simulink model "Filter"  (R2017b)
settings: Solver=VariableStepAuto  StartTime=0.0  StopTime=10  RelTol=1e-3
undefined symbols (not defined in the file or in its folder): designMultirateFIR
libraries: dspsrcs4 x2, dspmlti4 x1
(part 2 of 3)

== system Filter/HighpassH/Resonator132 ==
  In1 : Inport
  Delay : Delay  DelayLength=1
  Gain : Gain  Gain=-0.3143-0.94932i
  GainH : Gain  Gain=-0.57421+0.81871i
  Sum1 : Sum  Inputs=|++
  Out1 : Outport
  wires:
  In1/1 -> Sum1/1
  GainH/1 -> Out1/1
  Gain/1 -> Sum1/2
  Delay/1 -> Gain/1
  Sum1/1 -> Delay/1, GainH/1

== system Filter/HighpassH/Resonator133 ==
  In1 : Inport
  Delay : Delay  DelayLength=1
  Gain : Gain  Gain=-0.28779-0.95769i
  GainH : Gain  Gain=0.58553-0.81065i
  Sum1 : Sum  Inputs=|++
  Out1 : Outport
  wires:
  In1/1 -> Sum1/1
  GainH/1 -> Out1/1
  Gain/1 -> Sum1/2
  Delay/1 -> Gain/1
  Sum1/1 -> Delay/1, GainH/1

== system Filter/HighpassH/Resonator134 ==
  In1 : Inport
  Delay : Delay  DelayLength=1
  Gain : Gain  Gain=-0.26106-0.96532i
  GainH : Gain  Gain=-0.59675+0.80243i
  Sum1 : Sum  Inputs=|++
  Out1 : Outport
  wires:
  In1/1 -> Sum1/1
  GainH/1 -> Out1/1
  Gain/1 -> Sum1/2
  Delay/1 -> Gain/1
  Sum1/1 -> Delay/1, GainH/1

== system Filter/HighpassH/Resonator135 ==
  In1 : Inport
  Delay : Delay  DelayLength=1
  Gain : Gain  Gain=-0.23412-0.97221i
  GainH : Gain  Gain=0.60784-0.79406i
  Sum1 : Sum  Inputs=|++
  Out1 : Outport
  wires:
  In1/1 -> Sum1/1
  GainH/1 -> Out1/1
  Gain/1 -> Sum1/2
  Delay/1 -> Gain/1
  Sum1/1 -> Delay/1, GainH/1

== system Filter/HighpassH/Resonator136 ==
  In1 : Inport
  Delay : Delay  DelayLength=1
  Gain : Gain  Gain=-0.20701-0.97834i
  GainH : Gain  Gain=-0.61882+0.78553i
  Sum1 : Sum  Inputs=|++
  Out1 : Outport
  wires:
  In1/1 -> Sum1/1
  GainH/1 -> Out1/1
  Gain/1 -> Sum1/2
  Delay/1 -> Gain/1
  Sum1/1 -> Delay/1, GainH/1

== system Filter/HighpassH/Resonator137 ==
  In1 : Inport
  Delay : Delay  DelayLength=1
  Gain : Gain  Gain=-0.17973-0.98372i
  GainH : Gain  Gain=0.62968-0.77685i
  Sum1 : Sum  Inputs=|++
  Out1 : Outport
  wires:
  In1/1 -> Sum1/1
  GainH/1 -> Out1/1
  Gain/1 -> Sum1/2
  Delay/1 -> Gain/1
  Sum1/1 -> Delay/1, GainH/1

== system Filter/HighpassH/Resonator138 ==
  In1 : Inport
  Delay : Delay  DelayLength=1
  Gain : Gain  Gain=-0.15231-0.98833i
  GainH : Gain  Gain=-0.64042+0.76803i
  Sum1 : Sum  Inputs=|++
  Out1 : Outport
  wires:
  In1/1 -> Sum1/1
  GainH/1 -> Out1/1
  Gain/1 -> Sum1/2
  Delay/1 -> Gain/1
  Sum1/1 -> Delay/1, GainH/1

== system Filter/HighpassH/Resonator139 ==
  In1 : Inport
  Delay : Delay  DelayLength=1
  Gain : Gain  Gain=-0.12478-0.99218i
  GainH : Gain  Gain=0.65103-0.75905i
  Sum1 : Sum  Inputs=|++
  Out1 : Outport
  wires:
  In1/1 -> Sum1/1
  GainH/1 -> Out1/1
  Gain/1 -> Sum1/2
  Delay/1 -> Gain/1
  Sum1/1 -> Delay/1, GainH/1

== system Filter/HighpassH/Resonator14 ==
  In1 : Inport
  Delay : Delay  DelayLength=1
  Gain : Gain  Gain=0.44281+0.89662i
  GainH : Gain  Gain=-0.85661-0.51596i
  Sum1 : Sum  Inputs=|++
  Out1 : Outport
  wires:
  In1/1 -> Sum1/1
  GainH/1 -> Out1/1
  Gain/1 -> Sum1/2
  Delay/1 -> Gain/1
  Sum1/1 -> Delay/1, GainH/1

== system Filter/HighpassH/Resonator140 ==
  In1 : Inport
  Delay : Delay  DelayLength=1
  Gain : Gain  Gain=-0.097152-0.99527i
  GainH : Gain  Gain=-0.66152+0.74993i
  Sum1 : Sum  Inputs=|++
  Out1 : Outport
  wires:
  In1/1 -> Sum1/1
  GainH/1 -> Out1/1
  Gain/1 -> Sum1/2
  Delay/1 -> Gain/1
  Sum1/1 -> Delay/1, GainH/1

== system Filter/HighpassH/Resonator141 ==
  In1 : Inport
  Delay : Delay  DelayLength=1
  Gain : Gain  Gain=-0.069448-0.99759i
  GainH : Gain  Gain=0.67188-0.74066i
  Sum1 : Sum  Inputs=|++
  Out1 : Outport
  wires:
  In1/1 -> Sum1/1
  GainH/1 -> Out1/1
  Gain/1 -> Sum1/2
  Delay/1 -> Gain/1
  Sum1/1 -> Delay/1, GainH/1

== system Filter/HighpassH/Resonator142 ==
  In1 : Inport
  Delay : Delay  DelayLength=1
  Gain : Gain  Gain=-0.04169-0.99913i
  GainH : Gain  Gain=-0.68211+0.73125i
  Sum1 : Sum  Inputs=|++
  Out1 : Outport
  wires:
  In1/1 -> Sum1/1
  GainH/1 -> Out1/1
  Gain/1 -> Sum1/2
  Delay/1 -> Gain/1
  Sum1/1 -> Delay/1, GainH/1

== system Filter/HighpassH/Resonator143 ==
  In1 : Inport
  Delay : Delay  DelayLength=1
  Gain : Gain  Gain=-0.0139-0.9999i
  GainH : Gain  Gain=0.69221-0.7217i
  Sum1 : Sum  Inputs=|++
  Out1 : Outport
  wires:
  In1/1 -> Sum1/1
  GainH/1 -> Out1/1
  Gain/1 -> Sum1/2
  Delay/1 -> Gain/1
  Sum1/1 -> Delay/1, GainH/1

== system Filter/HighpassH/Resonator144 ==
  In1 : Inport
  Delay : Delay  DelayLength=1
  Gain : Gain  Gain=0.0139-0.9999i
  GainH : Gain  Gain=-0.70218+0.712i
  Sum1 : Sum  Inputs=|++
  Out1 : Outport
  wires:
  In1/1 -> Sum1/1
  GainH/1 -> Out1/1
  Gain/1 -> Sum1/2
  Delay/1 -> Gain/1
  Sum1/1 -> Delay/1, GainH/1

== system Filter/HighpassH/Resonator145 ==
  In1 : Inport
  Delay : Delay  DelayLength=1
  Gain : Gain  Gain=0.04169-0.99913i
  GainH : Gain  Gain=0.712-0.70218i
  Sum1 : Sum  Inputs=|++
  Out1 : Outport
  wires:
  In1/1 -> Sum1/1
  GainH/1 -> Out1/1
  Gain/1 -> Sum1/2
  Delay/1 -> Gain/1
  Sum1/1 -> Delay/1, GainH/1

== system Filter/HighpassH/Resonator146 ==
  In1 : Inport
  Delay : Delay  DelayLength=1
  Gain : Gain  Gain=0.069448-0.99759i
  GainH : Gain  Gain=-0.7217+0.69221i
  Sum1 : Sum  Inputs=|++
  Out1 : Outport
  wires:
  In1/1 -> Sum1/1
  GainH/1 -> Out1/1
  Gain/1 -> Sum1/2
  Delay/1 -> Gain/1
  Sum1/1 -> Delay/1, GainH/1

== system Filter/HighpassH/Resonator147 ==
  In1 : Inport
  Delay : Delay  DelayLength=1
  Gain : Gain  Gain=0.097152-0.99527i
  GainH : Gain  Gain=0.73125-0.68211i
  Sum1 : Sum  Inputs=|++
  Out1 : Outport
  wires:
  In1/1 -> Sum1/1
  GainH/1 -> Out1/1
  Gain/1 -> Sum1/2
  Delay/1 -> Gain/1
  Sum1/1 -> Delay/1, GainH/1

== system Filter/HighpassH/Resonator148 ==
  In1 : Inport
  Delay : Delay  DelayLength=1
  Gain : Gain  Gain=0.12478-0.99218i
  GainH : Gain  Gain=-0.74066+0.67188i
  Sum1 : Sum  Inputs=|++
  Out1 : Outport
  wires:
  In1/1 -> Sum1/1
  GainH/1 -> Out1/1
  Gain/1 -> Sum1/2
  Delay/1 -> Gain/1
  Sum1/1 -> Delay/1, GainH/1

== system Filter/HighpassH/Resonator149 ==
  In1 : Inport
  Delay : Delay  DelayLength=1
  Gain : Gain  Gain=0.15231-0.98833i
  GainH : Gain  Gain=0.74993-0.66152i
  Sum1 : Sum  Inputs=|++
  Out1 : Outport
  wires:
  In1/1 -> Sum1/1
  GainH/1 -> Out1/1
  Gain/1 -> Sum1/2
  Delay/1 -> Gain/1
  Sum1/1 -> Delay/1, GainH/1

== system Filter/HighpassH/Resonator15 ==
  In1 : Inport
  Delay : Delay  DelayLength=1
  Gain : Gain  Gain=0.41771+0.90858i
  GainH : Gain  Gain=0.84936+0.52782i
  Sum1 : Sum  Inputs=|++
  Out1 : Outport
  wires:
  In1/1 -> Sum1/1
  GainH/1 -> Out1/1
  Gain/1 -> Sum1/2
  Delay/1 -> Gain/1
  Sum1/1 -> Delay/1, GainH/1

== system Filter/HighpassH/Resonator150 ==
  In1 : Inport
  Delay : Delay  DelayLength=1
  Gain : Gain  Gain=0.17973-0.98372i
  GainH : Gain  Gain=-0.75905+0.65103i
  Sum1 : Sum  Inputs=|++
  Out1 : Outport
  wires:
  In1/1 -> Sum1/1
  GainH/1 -> Out1/1
  Gain/1 -> Sum1/2
  Delay/1 -> Gain/1
  Sum1/1 -> Delay/1, GainH/1

== system Filter/HighpassH/Resonator151 ==
  In1 : Inport
  Delay : Delay  DelayLength=1
  Gain : Gain  Gain=0.20701-0.97834i
  GainH : Gain  Gain=0.76803-0.64042i
  Sum1 : Sum  Inputs=|++
  Out1 : Outport
  wires:
  In1/1 -> Sum1/1
  GainH/1 -> Out1/1
  Gain/1 -> Sum1/2
  Delay/1 -> Gain/1
  Sum1/1 -> Delay/1, GainH/1

== system Filter/HighpassH/Resonator152 ==
  In1 : Inport
  Delay : Delay  DelayLength=1
  Gain : Gain  Gain=0.23412-0.97221i
  GainH : Gain  Gain=-0.77685+0.62968i
  Sum1 : Sum  Inputs=|++
  Out1 : Outport
  wires:
  In1/1 -> Sum1/1
  GainH/1 -> Out1/1
  Gain/1 -> Sum1/2
  Delay/1 -> Gain/1
  Sum1/1 -> Delay/1, GainH/1

== system Filter/HighpassH/Resonator153 ==
  In1 : Inport
  Delay : Delay  DelayLength=1
  Gain : Gain  Gain=0.26106-0.96532i
  GainH : Gain  Gain=0.78553-0.61882i
  Sum1 : Sum  Inputs=|++
  Out1 : Outport
  wires:
  In1/1 -> Sum1/1
  GainH/1 -> Out1/1
  Gain/1 -> Sum1/2
  Delay/1 -> Gain/1
  Sum1/1 -> Delay/1, GainH/1

== system Filter/HighpassH/Resonator154 ==
  In1 : Inport
  Delay : Delay  DelayLength=1
  Gain : Gain  Gain=0.28779-0.95769i
  GainH : Gain  Gain=-0.79406+0.60784i
  Sum1 : Sum  Inputs=|++
  Out1 : Outport
  wires:
  In1/1 -> Sum1/1
  GainH/1 -> Out1/1
  Gain/1 -> Sum1/2
  Delay/1 -> Gain/1
  Sum1/1 -> Delay/1, GainH/1

== system Filter/HighpassH/Resonator155 ==
  In1 : Inport
  Delay : Delay  DelayLength=1
  Gain : Gain  Gain=0.3143-0.94932i
  GainH : Gain  Gain=0.80243-0.59675i
  Sum1 : Sum  Inputs=|++
  Out1 : Outport
  wires:
  In1/1 -> Sum1/1
  GainH/1 -> Out1/1
  Gain/1 -> Sum1/2
  Delay/1 -> Gain/1
  Sum1/1 -> Delay/1, GainH/1

== system Filter/HighpassH/Resonator156 ==
  In1 : Inport
  Delay : Delay  DelayLength=1
  Gain : Gain  Gain=0.34057-0.94022i
  GainH : Gain  Gain=-0.81065+0.58553i
  Sum1 : Sum  Inputs=|++
  Out1 : Outport
  wires:
  In1/1 -> Sum1/1
  GainH/1 -> Out1/1
  Gain/1 -> Sum1/2
  Delay/1 -> Gain/1
  Sum1/1 -> Delay/1, GainH/1

== system Filter/HighpassH/Resonator157 ==
  In1 : Inport
  Delay : Delay  DelayLength=1
  Gain : Gain  Gain=0.36657-0.93039i
  GainH : Gain  Gain=0.81871-0.57421i
  Sum1 : Sum  Inputs=|++
  Out1 : Outport
  wires:
  In1/1 -> Sum1/1
  GainH/1 -> Out1/1
  Gain/1 -> Sum1/2
  Delay/1 -> Gain/1
  Sum1/1 -> Delay/1, GainH/1

== system Filter/HighpassH/Resonator158 ==
  In1 : Inport
  Delay : Delay  DelayLength=1
  Gain : Gain  Gain=0.39229-0.91984i
  GainH : Gain  Gain=-0.82661+0.56277i
  Sum1 : Sum  Inputs=|++
  Out1 : Outport
  wires:
  In1/1 -> Sum1/1
  GainH/1 -> Out1/1
  Gain/1 -> Sum1/2
  Delay/1 -> Gain/1
  Sum1/1 -> Delay/1, GainH/1

== system Filter/HighpassH/Resonator159 ==
  In1 : Inport
  Delay : Delay  DelayLength=1
  Gain : Gain  Gain=0.41771-0.90858i
  GainH : Gain  Gain=0.83435-0.55123i
  Sum1 : Sum  Inputs=|++
  Out1 : Outport
  wires:
  In1/1 -> Sum1/1
  GainH/1 -> Out1/1
  Gain/1 -> Sum1/2
  Delay/1 -> Gain/1
  Sum1/1 -> Delay/1, GainH/1

== system Filter/HighpassH/Resonator16 ==
  In1 : Inport
  Delay : Delay  DelayLength=1
  Gain : Gain  Gain=0.39229+0.91984i
  GainH : Gain  Gain=-0.84194-0.53958i
  Sum1 : Sum  Inputs=|++
  Out1 : Outport
  wires:
  In1/1 -> Sum1/1
  GainH/1 -> Out1/1
  Gain/1 -> Sum1/2
  Delay/1 -> Gain/1
  Sum1/1 -> Delay/1, GainH/1

== system Filter/HighpassH/Resonator160 ==
  In1 : Inport
  Delay : Delay  DelayLength=1
  Gain : Gain  Gain=0.44281-0.89662i
  GainH : Gain  Gain=-0.84194+0.53958i
  Sum1 : Sum  Inputs=|++
  Out1 : Outport
  wires:
  In1/1 -> Sum1/1
  GainH/1 -> Out1/1
  Gain/1 -> Sum1/2
  Delay/1 -> Gain/1
  Sum1/1 -> Delay/1, GainH/1

== system Filter/HighpassH/Resonator161 ==
  In1 : Inport
  Delay : Delay  DelayLength=1
  Gain : Gain  Gain=0.46756-0.88396i
  GainH : Gain  Gain=0.84936-0.52782i
  Sum1 : Sum  Inputs=|++
  Out1 : Outport
  wires:
  In1/1 -> Sum1/1
  GainH/1 -> Out1/1
  Gain/1 -> Sum1/2
  Delay/1 -> Gain/1
  Sum1/1 -> Delay/1, GainH/1

== system Filter/HighpassH/Resonator162 ==
  In1 : Inport
  Delay : Delay  DelayLength=1
  Gain : Gain  Gain=0.49195-0.87062i
  GainH : Gain  Gain=-0.85661+0.51596i
  Sum1 : Sum  Inputs=|++
  Out1 : Outport
  wires:
  In1/1 -> Sum1/1
  GainH/1 -> Out1/1
  Gain/1 -> Sum1/2
  Delay/1 -> Gain/1
  Sum1/1 -> Delay/1, GainH/1

== system Filter/HighpassH/Resonator163 ==
  In1 : Inport
  Delay : Delay  DelayLength=1
  Gain : Gain  Gain=0.51596-0.85661i
  GainH : Gain  Gain=0.8637-0.50401i
  Sum1 : Sum  Inputs=|++
  Out1 : Outport
  wires:
  In1/1 -> Sum1/1
  GainH/1 -> Out1/1
  Gain/1 -> Sum1/2
  Delay/1 -> Gain/1
  Sum1/1 -> Delay/1, GainH/1

== system Filter/HighpassH/Resonator164 ==
  In1 : Inport
  Delay : Delay  DelayLength=1
  Gain : Gain  Gain=0.53958-0.84194i
  GainH : Gain  Gain=-0.87062+0.49195i
  Sum1 : Sum  Inputs=|++
  Out1 : Outport
  wires:
  In1/1 -> Sum1/1
  GainH/1 -> Out1/1
  Gain/1 -> Sum1/2
  Delay/1 -> Gain/1
  Sum1/1 -> Delay/1, GainH/1

== system Filter/HighpassH/Resonator165 ==
  In1 : Inport
  Delay : Delay  DelayLength=1
  Gain : Gain  Gain=0.56277-0.82661i
  GainH : Gain  Gain=0.87738-0.4798i
  Sum1 : Sum  Inputs=|++
  Out1 : Outport
  wires:
  In1/1 -> Sum1/1
  GainH/1 -> Out1/1
  Gain/1 -> Sum1/2
  Delay/1 -> Gain/1
  Sum1/1 -> Delay/1, GainH/1

== system Filter/HighpassH/Resonator166 ==
  In1 : Inport
  Delay : Delay  DelayLength=1
  Gain : Gain  Gain=0.58553-0.81065i
  GainH : Gain  Gain=-0.88396+0.46756i
  Sum1 : Sum  Inputs=|++
  Out1 : Outport
  wires:
  In1/1 -> Sum1/1
  GainH/1 -> Out1/1
  Gain/1 -> Sum1/2
  Delay/1 -> Gain/1
  Sum1/1 -> Delay/1, GainH/1

== system Filter/HighpassH/Resonator167 ==
  In1 : Inport
  Delay : Delay  DelayLength=1
  Gain : Gain  Gain=0.60784-0.79406i
  GainH : Gain  Gain=0.89037-0.45523i
  Sum1 : Sum  Inputs=|++
  Out1 : Outport
  wires:
  In1/1 -> Sum1/1
  GainH/1 -> Out1/1
  Gain/1 -> Sum1/2
  Delay/1 -> Gain/1
  Sum1/1 -> Delay/1, GainH/1

== system Filter/HighpassH/Resonator168 ==
  In1 : Inport
  Delay : Delay  DelayLength=1
  Gain : Gain  Gain=0.62968-0.77685i
  GainH : Gain  Gain=-0.89662+0.44281i
  Sum1 : Sum  Inputs=|++
  Out1 : Outport
  wires:
  In1/1 -> Sum1/1
  GainH/1 -> Out1/1
  Gain/1 -> Sum1/2
  Delay/1 -> Gain/1
  Sum1/1 -> Delay/1, GainH/1

== system Filter/HighpassH/Resonator169 ==
  In1 : Inport
  Delay : Delay  DelayLength=1
  Gain : Gain  Gain=0.65103-0.75905i
  GainH : Gain  Gain=0.90269-0.4303i
  Sum1 : Sum  Inputs=|++
  Out1 : Outport
  wires:
  In1/1 -> Sum1/1
  GainH/1 -> Out1/1
  Gain/1 -> Sum1/2
  Delay/1 -> Gain/1
  Sum1/1 -> Delay/1, GainH/1

== system Filter/HighpassH/Resonator17 ==
  In1 : Inport
  Delay : Delay  DelayLength=1
  Gain : Gain  Gain=0.36657+0.93039i
  GainH : Gain  Gain=0.83435+0.55123i
  Sum1 : Sum  Inputs=|++
  Out1 : Outport
  wires:
  In1/1 -> Sum1/1
  GainH/1 -> Out1/1
  Gain/1 -> Sum1/2
  Delay/1 -> Gain/1
  Sum1/1 -> Delay/1, GainH/1

== system Filter/HighpassH/Resonator170 ==
  In1 : Inport
  Delay : Delay  DelayLength=1
  Gain : Gain  Gain=0.67188-0.74066i
  GainH : Gain  Gain=-0.90858+0.41771i
  Sum1 : Sum  Inputs=|++
  Out1 : Outport
  wires:
  In1/1 -> Sum1/1
  GainH/1 -> Out1/1
  Gain/1 -> Sum1/2
  Delay/1 -> Gain/1
  Sum1/1 -> Delay/1, GainH/1

== system Filter/HighpassH/Resonator171 ==
  In1 : Inport
  Delay : Delay  DelayLength=1
  Gain : Gain  Gain=0.69221-0.7217i
  GainH : Gain  Gain=0.9143-0.40504i
  Sum1 : Sum  Inputs=|++
  Out1 : Outport
  wires:
  In1/1 -> Sum1/1
  GainH/1 -> Out1/1
  Gain/1 -> Sum1/2
  Delay/1 -> Gain/1
  Sum1/1 -> Delay/1, GainH/1

== system Filter/HighpassH/Resonator172 ==
  In1 : Inport
  Delay : Delay  DelayLength=1
  Gain : Gain  Gain=0.712-0.70218i
  GainH : Gain  Gain=-0.91984+0.39229i
  Sum1 : Sum  Inputs=|++
  Out1 : Outport
  wires:
  In1/1 -> Sum1/1
  GainH/1 -> Out1/1
  Gain/1 -> Sum1/2
  Delay/1 -> Gain/1
  Sum1/1 -> Delay/1, GainH/1

== system Filter/HighpassH/Resonator173 ==
  In1 : Inport
  Delay : Delay  DelayLength=1
  Gain : Gain  Gain=0.73125-0.68211i
  GainH : Gain  Gain=0.9252-0.37947i
  Sum1 : Sum  Inputs=|++
  Out1 : Outport
  wires:
  In1/1 -> Sum1/1
  GainH/1 -> Out1/1
  Gain/1 -> Sum1/2
  Delay/1 -> Gain/1
  Sum1/1 -> Delay/1, GainH/1

== system Filter/HighpassH/Resonator174 ==
  In1 : Inport
  Delay : Delay  DelayLength=1
  Gain : Gain  Gain=0.74993-0.66152i
  GainH : Gain  Gain=-0.93039+0.36657i
  Sum1 : Sum  Inputs=|++
  Out1 : Outport
  wires:
  In1/1 -> Sum1/1
  GainH/1 -> Out1/1
  Gain/1 -> Sum1/2
  Delay/1 -> Gain/1
  Sum1/1 -> Delay/1, GainH/1

== system Filter/HighpassH/Resonator175 ==
  In1 : Inport
  Delay : Delay  DelayLength=1
  Gain : Gain  Gain=0.76803-0.64042i
  GainH : Gain  Gain=0.93539-0.3536i
  Sum1 : Sum  Inputs=|++
  Out1 : Outport
  wires:
  In1/1 -> Sum1/1
  GainH/1 -> Out1/1
  Gain/1 -> Sum1/2
  Delay/1 -> Gain/1
  Sum1/1 -> Delay/1, GainH/1

== system Filter/HighpassH/Resonator18 ==
  In1 : Inport
  Delay : Delay  DelayLength=1
  Gain : Gain  Gain=0.34057+0.94022i
  GainH : Gain  Gain=-0.82661-0.56277i
  Sum1 : Sum  Inputs=|++
  Out1 : Outport
  wires:
  In1/1 -> Sum1/1
  GainH/1 -> Out1/1
  Gain/1 -> Sum1/2
  Delay/1 -> Gain/1
  Sum1/1 -> Delay/1, GainH/1

== system Filter/HighpassH/Resonator19 ==
  In1 : Inport
  Delay : Delay  DelayLength=1
  Gain : Gain  Gain=0.3143+0.94932i
  GainH : Gain  Gain=0.81871+0.57421i
  Sum1 : Sum  Inputs=|++
  Out1 : Outport
  wires:
  In1/1 -> Sum1/1
  GainH/1 -> Out1/1
  Gain/1 -> Sum1/2
  Delay/1 -> Gain/1
  Sum1/1 -> Delay/1, GainH/1

== system Filter/HighpassH/Resonator2 ==
  In1 : Inport
  Delay : Delay  DelayLength=1
  Gain : Gain  Gain=0.712+0.70218i
  GainH : Gain  Gain=-0.93039-0.36657i
  Sum1 : Sum  Inputs=|++
  Out1 : Outport
  wires:
  In1/1 -> Sum1/1
  GainH/1 -> Out1/1
  Gain/1 -> Sum1/2
  Delay/1 -> Gain/1
  Sum1/1 -> Delay/1, GainH/1

== system Filter/HighpassH/Resonator20 ==
  In1 : Inport
  Delay : Delay  DelayLength=1
  Gain : Gain  Gain=0.28779+0.95769i
  GainH : Gain  Gain=-0.81065-0.58553i
  Sum1 : Sum  Inputs=|++
  Out1 : Outport
  wires:
  In1/1 -> Sum1/1
  GainH/1 -> Out1/1
  Gain/1 -> Sum1/2
  Delay/1 -> Gain/1
  Sum1/1 -> Delay/1, GainH/1

== system Filter/HighpassH/Resonator21 ==
  In1 : Inport
  Delay : Delay  DelayLength=1
  Gain : Gain  Gain=0.26106+0.96532i
  GainH : Gain  Gain=0.80243+0.59675i
  Sum1 : Sum  Inputs=|++
  Out1 : Outport
  wires:
  In1/1 -> Sum1/1
  GainH/1 -> Out1/1
  Gain/1 -> Sum1/2
  Delay/1 -> Gain/1
  Sum1/1 -> Delay/1, GainH/1

== system Filter/HighpassH/Resonator22 ==
  In1 : Inport
  Delay : Delay  DelayLength=1
  Gain : Gain  Gain=0.23412+0.97221i
  GainH : Gain  Gain=-0.79406-0.60784i
  Sum1 : Sum  Inputs=|++
  Out1 : Outport
  wires:
  In1/1 -> Sum1/1
  GainH/1 -> Out1/1
  Gain/1 -> Sum1/2
  Delay/1 -> Gain/1
  Sum1/1 -> Delay/1, GainH/1

== system Filter/HighpassH/Resonator23 ==
  In1 : Inport
  Delay : Delay  DelayLength=1
  Gain : Gain  Gain=0.20701+0.97834i
  GainH : Gain  Gain=0.78553+0.61882i
  Sum1 : Sum  Inputs=|++
  Out1 : Outport
  wires:
  In1/1 -> Sum1/1
  GainH/1 -> Out1/1
  Gain/1 -> Sum1/2
  Delay/1 -> Gain/1
  Sum1/1 -> Delay/1, GainH/1

== system Filter/HighpassH/Resonator24 ==
  In1 : Inport
  Delay : Delay  DelayLength=1
  Gain : Gain  Gain=0.17973+0.98372i
  GainH : Gain  Gain=-0.77685-0.62968i
  Sum1 : Sum  Inputs=|++
  Out1 : Outport
  wires:
  In1/1 -> Sum1/1
  GainH/1 -> Out1/1
  Gain/1 -> Sum1/2
  Delay/1 -> Gain/1
  Sum1/1 -> Delay/1, GainH/1

== system Filter/HighpassH/Resonator25 ==
  In1 : Inport
  Delay : Delay  DelayLength=1
  Gain : Gain  Gain=0.15231+0.98833i
  GainH : Gain  Gain=0.76803+0.64042i
  Sum1 : Sum  Inputs=|++
  Out1 : Outport
  wires:
  In1/1 -> Sum1/1
  GainH/1 -> Out1/1
  Gain/1 -> Sum1/2
  Delay/1 -> Gain/1
  Sum1/1 -> Delay/1, GainH/1

== system Filter/HighpassH/Resonator26 ==
  In1 : Inport
  Delay : Delay  DelayLength=1
  Gain : Gain  Gain=0.12478+0.99218i
  GainH : Gain  Gain=-0.75905-0.65103i
  Sum1 : Sum  Inputs=|++
  Out1 : Outport
  wires:
  In1/1 -> Sum1/1
  GainH/1 -> Out1/1
  Gain/1 -> Sum1/2
  Delay/1 -> Gain/1
  Sum1/1 -> Delay/1, GainH/1

== system Filter/HighpassH/Resonator27 ==
  In1 : Inport
  Delay : Delay  DelayLength=1
  Gain : Gain  Gain=0.097152+0.99527i
  GainH : Gain  Gain=0.74993+0.66152i
  Sum1 : Sum  Inputs=|++
  Out1 : Outport
  wires:
  In1/1 -> Sum1/1
  GainH/1 -> Out1/1
  Gain/1 -> Sum1/2
  Delay/1 -> Gain/1
  Sum1/1 -> Delay/1, GainH/1

== system Filter/HighpassH/Resonator28 ==
  In1 : Inport
  Delay : Delay  DelayLength=1
  Gain : Gain  Gain=0.069448+0.99759i
  GainH : Gain  Gain=-0.74066-0.67188i
  Sum1 : Sum  Inputs=|++
  Out1 : Outport
  wires:
  In1/1 -> Sum1/1
  GainH/1 -> Out1/1
  Gain/1 -> Sum1/2
  Delay/1 -> Gain/1
  Sum1/1 -> Delay/1, GainH/1

== system Filter/HighpassH/Resonator29 ==
  In1 : Inport
  Delay : Delay  DelayLength=1
  Gain : Gain  Gain=0.04169+0.99913i
  GainH : Gain  Gain=0.73125+0.68211i
  Sum1 : Sum  Inputs=|++
  Out1 : Outport
  wires:
  In1/1 -> Sum1/1
  GainH/1 -> Out1/1
  Gain/1 -> Sum1/2
  Delay/1 -> Gain/1
  Sum1/1 -> Delay/1, GainH/1

== system Filter/HighpassH/Resonator3 ==
  In1 : Inport
  Delay : Delay  DelayLength=1
  Gain : Gain  Gain=0.69221+0.7217i
  GainH : Gain  Gain=0.9252+0.37947i
  Sum1 : Sum  Inputs=|++
  Out1 : Outport
  wires:
  In1/1 -> Sum1/1
  GainH/1 -> Out1/1
  Gain/1 -> Sum1/2
  Delay/1 -> Gain/1
  Sum1/1 -> Delay/1, GainH/1

== system Filter/HighpassH/Resonator30 ==
  In1 : Inport
  Delay : Delay  DelayLength=1
  Gain : Gain  Gain=0.0139+0.9999i
  GainH : Gain  Gain=-0.7217-0.69221i
  Sum1 : Sum  Inputs=|++
  Out1 : Outport
  wires:
  In1/1 -> Sum1/1
  GainH/1 -> Out1/1
  Gain/1 -> Sum1/2
  Delay/1 -> Gain/1
  Sum1/1 -> Delay/1, GainH/1

== system Filter/HighpassH/Resonator31 ==
  In1 : Inport
  Delay : Delay  DelayLength=1
  Gain : Gain  Gain=-0.0139+0.9999i
  GainH : Gain  Gain=0.712+0.70218i
  Sum1 : Sum  Inputs=|++
  Out1 : Outport
  wires:
  In1/1 -> Sum1/1
  GainH/1 -> Out1/1
  Gain/1 -> Sum1/2
  Delay/1 -> Gain/1
  Sum1/1 -> Delay/1, GainH/1

== system Filter/HighpassH/Resonator32 ==
  In1 : Inport
  Delay : Delay  DelayLength=1
  Gain : Gain  Gain=-0.04169+0.99913i
  GainH : Gain  Gain=-0.70218-0.712i
  Sum1 : Sum  Inputs=|++
  Out1 : Outport
  wires:
  In1/1 -> Sum1/1
  GainH/1 -> Out1/1
  Gain/1 -> Sum1/2
  Delay/1 -> Gain/1
  Sum1/1 -> Delay/1, GainH/1

== system Filter/HighpassH/Resonator33 ==
  In1 : Inport
  Delay : Delay  DelayLength=1
  Gain : Gain  Gain=-0.069448+0.99759i
  GainH : Gain  Gain=0.69221+0.7217i
  Sum1 : Sum  Inputs=|++
  Out1 : Outport
  wires:
  In1/1 -> Sum1/1
  GainH/1 -> Out1/1
  Gain/1 -> Sum1/2
  Delay/1 -> Gain/1
  Sum1/1 -> Delay/1, GainH/1

== system Filter/HighpassH/Resonator34 ==
  In1 : Inport
  Delay : Delay  DelayLength=1
  Gain : Gain  Gain=-0.097152+0.99527i
  GainH : Gain  Gain=-0.68211-0.73125i
  Sum1 : Sum  Inputs=|++
  Out1 : Outport
  wires:
  In1/1 -> Sum1/1
  GainH/1 -> Out1/1
  Gain/1 -> Sum1/2
  Delay/1 -> Gain/1
  Sum1/1 -> Delay/1, GainH/1

== system Filter/HighpassH/Resonator35 ==
  In1 : Inport
  Delay : Delay  DelayLength=1
  Gain : Gain  Gain=-0.12478+0.99218i
  GainH : Gain  Gain=0.67188+0.74066i
  Sum1 : Sum  Inputs=|++
  Out1 : Outport
  wires:
  In1/1 -> Sum1/1
  GainH/1 -> Out1/1
  Gain/1 -> Sum1/2
  Delay/1 -> Gain/1
  Sum1/1 -> Delay/1, GainH/1

== system Filter/HighpassH/Resonator36 ==
  In1 : Inport
  Delay : Delay  DelayLength=1
  Gain : Gain  Gain=-0.15231+0.98833i
  GainH : Gain  Gain=-0.66152-0.74993i
  Sum1 : Sum  Inputs=|++
  Out1 : Outport
  wires:
  In1/1 -> Sum1/1
  GainH/1 -> Out1/1
  Gain/1 -> Sum1/2
  Delay/1 -> Gain/1
  Sum1/1 -> Delay/1, GainH/1

== system Filter/HighpassH/Resonator37 ==
  In1 : Inport
  Delay : Delay  DelayLength=1
  Gain : Gain  Gain=-0.17973+0.98372i
  GainH : Gain  Gain=0.65103+0.75905i
  Sum1 : Sum  Inputs=|++
  Out1 : Outport
  wires:
  In1/1 -> Sum1/1
  GainH/1 -> Out1/1
  Gain/1 -> Sum1/2
  Delay/1 -> Gain/1
  Sum1/1 -> Delay/1, GainH/1

== system Filter/HighpassH/Resonator38 ==
  In1 : Inport
  Delay : Delay  DelayLength=1
  Gain : Gain  Gain=-0.20701+0.97834i
  GainH : Gain  Gain=-0.64042-0.76803i
  Sum1 : Sum  Inputs=|++
  Out1 : Outport
  wires:
  In1/1 -> Sum1/1
  GainH/1 -> Out1/1
  Gain/1 -> Sum1/2
  Delay/1 -> Gain/1
  Sum1/1 -> Delay/1, GainH/1

== system Filter/HighpassH/Resonator39 ==
  In1 : Inport
  Delay : Delay  DelayLength=1
  Gain : Gain  Gain=-0.23412+0.97221i
  GainH : Gain  Gain=0.62968+0.77685i
  Sum1 : Sum  Inputs=|++
  Out1 : Outport
  wires:
  In1/1 -> Sum1/1
  GainH/1 -> Out1/1
  Gain/1 -> Sum1/2
  Delay/1 -> Gain/1
  Sum1/1 -> Delay/1, GainH/1

== system Filter/HighpassH/Resonator4 ==
  In1 : Inport
  Delay : Delay  DelayLength=1
  Gain : Gain  Gain=0.67188+0.74066i
  GainH : Gain  Gain=-0.91984-0.39229i
  Sum1 : Sum  Inputs=|++
  Out1 : Outport
  wires:
  In1/1 -> Sum1/1
  GainH/1 -> Out1/1
  Gain/1 -> Sum1/2
  Delay/1 -> Gain/1
  Sum1/1 -> Delay/1, GainH/1

== system Filter/HighpassH/Resonator40 ==
  In1 : Inport
  Delay : Delay  DelayLength=1
  Gain : Gain  Gain=-0.26106+0.96532i
  GainH : Gain  Gain=-0.61882-0.78553i
  Sum1 : Sum  Inputs=|++
  Out1 : Outport
  wires:
  In1/1 -> Sum1/1
  GainH/1 -> Out1/1
  Gain/1 -> Sum1/2
  Delay/1 -> Gain/1
  Sum1/1 -> Delay/1, GainH/1

== system Filter/HighpassH/Resonator41 ==
  In1 : Inport
  Delay : Delay  DelayLength=1
  Gain : Gain  Gain=-0.28779+0.95769i
  GainH : Gain  Gain=0.60784+0.79406i
  Sum1 : Sum  Inputs=|++
  Out1 : Outport
  wires:
  In1/1 -> Sum1/1
  GainH/1 -> Out1/1
  Gain/1 -> Sum1/2
  Delay/1 -> Gain/1
  Sum1/1 -> Delay/1, GainH/1

== system Filter/HighpassH/Resonator42 ==
  In1 : Inport
  Delay : Delay  DelayLength=1
  Gain : Gain  Gain=-0.3143+0.94932i
  GainH : Gain  Gain=-0.59675-0.80243i
  Sum1 : Sum  Inputs=|++
  Out1 : Outport
  wires:
  In1/1 -> Sum1/1
  GainH/1 -> Out1/1
  Gain/1 -> Sum1/2
  Delay/1 -> Gain/1
  Sum1/1 -> Delay/1, GainH/1

== system Filter/HighpassH/Resonator43 ==
  In1 : Inport
  Delay : Delay  DelayLength=1
  Gain : Gain  Gain=-0.34057+0.94022i
  GainH : Gain  Gain=0.58553+0.81065i
  Sum1 : Sum  Inputs=|++
  Out1 : Outport
  wires:
  In1/1 -> Sum1/1
  GainH/1 -> Out1/1
  Gain/1 -> Sum1/2
  Delay/1 -> Gain/1
  Sum1/1 -> Delay/1, GainH/1

== system Filter/HighpassH/Resonator44 ==
  In1 : Inport
  Delay : Delay  DelayLength=1
  Gain : Gain  Gain=-0.36657+0.93039i
  GainH : Gain  Gain=-0.57421-0.81871i
  Sum1 : Sum  Inputs=|++
  Out1 : Outport
  wires:
  In1/1 -> Sum1/1
  GainH/1 -> Out1/1
  Gain/1 -> Sum1/2
  Delay/1 -> Gain/1
  Sum1/1 -> Delay/1, GainH/1

== system Filter/HighpassH/Resonator45 ==
  In1 : Inport
  Delay : Delay  DelayLength=1
  Gain : Gain  Gain=-0.39229+0.91984i
  GainH : Gain  Gain=0.56277+0.82661i
  Sum1 : Sum  Inputs=|++
  Out1 : Outport
  wires:
  In1/1 -> Sum1/1
  GainH/1 -> Out1/1
  Gain/1 -> Sum1/2
  Delay/1 -> Gain/1
  Sum1/1 -> Delay/1, GainH/1

== system Filter/HighpassH/Resonator46 ==
  In1 : Inport
  Delay : Delay  DelayLength=1
  Gain : Gain  Gain=-0.41771+0.90858i
  GainH : Gain  Gain=-0.55123-0.83435i
  Sum1 : Sum  Inputs=|++
  Out1 : Outport
  wires:
  In1/1 -> Sum1/1
  GainH/1 -> Out1/1
  Gain/1 -> Sum1/2
  Delay/1 -> Gain/1
  Sum1/1 -> Delay/1, GainH/1

== system Filter/HighpassH/Resonator47 ==
  In1 : Inport
  Delay : Delay  DelayLength=1
  Gain : Gain  Gain=-0.44281+0.89662i
  GainH : Gain  Gain=0.53958+0.84194i
  Sum1 : Sum  Inputs=|++
  Out1 : Outport
  wires:
  In1/1 -> Sum1/1
  GainH/1 -> Out1/1
  Gain/1 -> Sum1/2
  Delay/1 -> Gain/1
  Sum1/1 -> Delay/1, GainH/1

== system Filter/HighpassH/Resonator48 ==
  In1 : Inport
  Delay : Delay  DelayLength=1
  Gain : Gain  Gain=-0.46756+0.88396i
  GainH : Gain  Gain=-0.52782-0.84936i
  Sum1 : Sum  Inputs=|++
  Out1 : Outport
  wires:
  In1/1 -> Sum1/1
  GainH/1 -> Out1/1
  Gain/1 -> Sum1/2
  Delay/1 -> Gain/1
  Sum1/1 -> Delay/1, GainH/1

== system Filter/HighpassH/Resonator49 ==
  In1 : Inport
  Delay : Delay  DelayLength=1
  Gain : Gain  Gain=-0.49195+0.87062i
  GainH : Gain  Gain=0.51596+0.85661i
  Sum1 : Sum  Inputs=|++
  Out1 : Outport
  wires:
  In1/1 -> Sum1/1
  GainH/1 -> Out1/1
  Gain/1 -> Sum1/2
  Delay/1 -> Gain/1
  Sum1/1 -> Delay/1, GainH/1

== system Filter/HighpassH/Resonator5 ==
  In1 : Inport
  Delay : Delay  DelayLength=1
  Gain : Gain  Gain=0.65103+0.75905i
  GainH : Gain  Gain=0.9143+0.40504i
  Sum1 : Sum  Inputs=|++
  Out1 : Outport
  wires:
  In1/1 -> Sum1/1
  GainH/1 -> Out1/1
  Gain/1 -> Sum1/2
  Delay/1 -> Gain/1
  Sum1/1 -> Delay/1, GainH/1

== system Filter/HighpassH/Resonator50 ==
  In1 : Inport
  Delay : Delay  DelayLength=1
  Gain : Gain  Gain=-0.51596+0.85661i
  GainH : Gain  Gain=-0.50401-0.8637i
  Sum1 : Sum  Inputs=|++
  Out1 : Outport
  wires:
  In1/1 -> Sum1/1
  GainH/1 -> Out1/1
  Gain/1 -> Sum1/2
  Delay/1 -> Gain/1
  Sum1/1 -> Delay/1, GainH/1

== system Filter/HighpassH/Resonator51 ==
  In1 : Inport
  Delay : Delay  DelayLength=1
  Gain : Gain  Gain=-0.53958+0.84194i
  GainH : Gain  Gain=0.49195+0.87062i
  Sum1 : Sum  Inputs=|++
  Out1 : Outport
  wires:
  In1/1 -> Sum1/1
  GainH/1 -> Out1/1
  Gain/1 -> Sum1/2
  Delay/1 -> Gain/1
  Sum1/1 -> Delay/1, GainH/1

== system Filter/HighpassH/Resonator52 ==
  In1 : Inport
  Delay : Delay  DelayLength=1
  Gain : Gain  Gain=-0.56277+0.82661i
  GainH : Gain  Gain=-0.4798-0.87738i
  Sum1 : Sum  Inputs=|++
  Out1 : Outport
  wires:
  In1/1 -> Sum1/1
  GainH/1 -> Out1/1
  Gain/1 -> Sum1/2
  Delay/1 -> Gain/1
  Sum1/1 -> Delay/1, GainH/1

== system Filter/HighpassH/Resonator53 ==
  In1 : Inport
  Delay : Delay  DelayLength=1
  Gain : Gain  Gain=-0.58553+0.81065i
  GainH : Gain  Gain=0.46756+0.88396i
  Sum1 : Sum  Inputs=|++
  Out1 : Outport
  wires:
  In1/1 -> Sum1/1
  GainH/1 -> Out1/1
  Gain/1 -> Sum1/2
  Delay/1 -> Gain/1
  Sum1/1 -> Delay/1, GainH/1

== system Filter/HighpassH/Resonator54 ==
  In1 : Inport
  Delay : Delay  DelayLength=1
  Gain : Gain  Gain=-0.60784+0.79406i
  GainH : Gain  Gain=-0.45523-0.89037i
  Sum1 : Sum  Inputs=|++
  Out1 : Outport
  wires:
  In1/1 -> Sum1/1
  GainH/1 -> Out1/1
  Gain/1 -> Sum1/2
  Delay/1 -> Gain/1
  Sum1/1 -> Delay/1, GainH/1

== system Filter/HighpassH/Resonator55 ==
  In1 : Inport
  Delay : Delay  DelayLength=1
  Gain : Gain  Gain=-0.62968+0.77685i
  GainH : Gain  Gain=0.44281+0.89662i
  Sum1 : Sum  Inputs=|++
  Out1 : Outport
  wires:
  In1/1 -> Sum1/1
  GainH/1 -> Out1/1
  Gain/1 -> Sum1/2
  Delay/1 -> Gain/1
  Sum1/1 -> Delay/1, GainH/1

== system Filter/HighpassH/Resonator56 ==
  In1 : Inport
  Delay : Delay  DelayLength=1
  Gain : Gain  Gain=-0.65103+0.75905i
  GainH : Gain  Gain=-0.4303-0.90269i
  Sum1 : Sum  Inputs=|++
  Out1 : Outport
  wires:
  In1/1 -> Sum1/1
  GainH/1 -> Out1/1
  Gain/1 -> Sum1/2
  Delay/1 -> Gain/1
  Sum1/1 -> Delay/1, GainH/1

== system Filter/HighpassH/Resonator57 ==
  In1 : Inport
  Delay : Delay  DelayLength=1
  Gain : Gain  Gain=-0.67188+0.74066i
  GainH : Gain  Gain=0.41771+0.90858i
  Sum1 : Sum  Inputs=|++
  Out1 : Outport
  wires:
  In1/1 -> Sum1/1
  GainH/1 -> Out1/1
  Gain/1 -> Sum1/2
  Delay/1 -> Gain/1
  Sum1/1 -> Delay/1, GainH/1

== system Filter/HighpassH/Resonator58 ==
  In1 : Inport
  Delay : Delay  DelayLength=1
  Gain : Gain  Gain=-0.69221+0.7217i
  GainH : Gain  Gain=-0.40504-0.9143i
  Sum1 : Sum  Inputs=|++
  Out1 : Outport
  wires:
  In1/1 -> Sum1/1
  GainH/1 -> Out1/1
  Gain/1 -> Sum1/2
  Delay/1 -> Gain/1
  Sum1/1 -> Delay/1, GainH/1

== system Filter/HighpassH/Resonator59 ==
  In1 : Inport
  Delay : Delay  DelayLength=1
  Gain : Gain  Gain=-0.712+0.70218i
  GainH : Gain  Gain=0.39229+0.91984i
  Sum1 : Sum  Inputs=|++
  Out1 : Outport
  wires:
  In1/1 -> Sum1/1
  GainH/1 -> Out1/1
  Gain/1 -> Sum1/2
  Delay/1 -> Gain/1
  Sum1/1 -> Delay/1, GainH/1

== system Filter/HighpassH/Resonator6 ==
  In1 : Inport
  Delay : Delay  DelayLength=1
  Gain : Gain  Gain=0.62968+0.77685i
  GainH : Gain  Gain=-0.90858-0.41771i
  Sum1 : Sum  Inputs=|++
  Out1 : Outport
  wires:
  In1/1 -> Sum1/1
  GainH/1 -> Out1/1
  Gain/1 -> Sum1/2
  Delay/1 -> Gain/1
  Sum1/1 -> Delay/1, GainH/1

== system Filter/HighpassH/Resonator60 ==
  In1 : Inport
  Delay : Delay  DelayLength=1
  Gain : Gain  Gain=-0.73125+0.68211i
  GainH : Gain  Gain=-0.37947-0.9252i
  Sum1 : Sum  Inputs=|++
  Out1 : Outport
  wires:
  In1/1 -> Sum1/1
  GainH/1 -> Out1/1
  Gain/1 -> Sum1/2
  Delay/1 -> Gain/1
  Sum1/1 -> Delay/1, GainH/1

== system Filter/HighpassH/Resonator61 ==
  In1 : Inport
  Delay : Delay  DelayLength=1
  Gain : Gain  Gain=-0.74993+0.66152i
  GainH : Gain  Gain=0.36657+0.93039i
  Sum1 : Sum  Inputs=|++
  Out1 : Outport
  wires:
  In1/1 -> Sum1/1
  GainH/1 -> Out1/1
  Gain/1 -> Sum1/2
  Delay/1 -> Gain/1
  Sum1/1 -> Delay/1, GainH/1

== system Filter/HighpassH/Resonator62 ==
  In1 : Inport
  Delay : Delay  DelayLength=1
  Gain : Gain  Gain=-0.76803+0.64042i
  GainH : Gain  Gain=-0.3536-0.93539i
  Sum1 : Sum  Inputs=|++
  Out1 : Outport
  wires:
  In1/1 -> Sum1/1
  GainH/1 -> Out1/1
  Gain/1 -> Sum1/2
  Delay/1 -> Gain/1
  Sum1/1 -> Delay/1, GainH/1

== system Filter/HighpassH/Resonator63 ==
  In1 : Inport
  Delay : Delay  DelayLength=1
  Gain : Gain  Gain=-0.78553+0.61882i
  GainH : Gain  Gain=0.34057+0.94022i
  Sum1 : Sum  Inputs=|++
  Out1 : Outport
  wires:
  In1/1 -> Sum1/1
  GainH/1 -> Out1/1
  Gain/1 -> Sum1/2
  Delay/1 -> Gain/1
  Sum1/1 -> Delay/1, GainH/1

== system Filter/HighpassH/Resonator64 ==
  In1 : Inport
  Delay : Delay  DelayLength=1
  Gain : Gain  Gain=-0.80243+0.59675i
  GainH : Gain  Gain=-0.32747-0.94486i
  Sum1 : Sum  Inputs=|++
  Out1 : Outport
  wires:
  In1/1 -> Sum1/1
  GainH/1 -> Out1/1
  Gain/1 -> Sum1/2
  Delay/1 -> Gain/1
  Sum1/1 -> Delay/1, GainH/1

== system Filter/HighpassH/Resonator65 ==
  In1 : Inport
  Delay : Delay  DelayLength=1
  Gain : Gain  Gain=-0.81871+0.57421i
  GainH : Gain  Gain=0.3143+0.94932i
  Sum1 : Sum  Inputs=|++
  Out1 : Outport
  wires:
  In1/1 -> Sum1/1
  GainH/1 -> Out1/1
  Gain/1 -> Sum1/2
  Delay/1 -> Gain/1
  Sum1/1 -> Delay/1, GainH/1

== system Filter/HighpassH/Resonator66 ==
  In1 : Inport
  Delay : Delay  DelayLength=1
  Gain : Gain  Gain=-0.83435+0.55123i
  GainH : Gain  Gain=-0.30107-0.9536i
  Sum1 : Sum  Inputs=|++
  Out1 : Outport
  wires:
  In1/1 -> Sum1/1
  GainH/1 -> Out1/1
  Gain/1 -> Sum1/2
  Delay/1 -> Gain/1
  Sum1/1 -> Delay/1, GainH/1

== system Filter/HighpassH/Resonator67 ==
  In1 : Inport
  Delay : Delay  DelayLength=1
  Gain : Gain  Gain=-0.84936+0.52782i
  GainH : Gain  Gain=0.28779+0.95769i
  Sum1 : Sum  Inputs=|++
  Out1 : Outport
  wires:
  In1/1 -> Sum1/1
  GainH/1 -> Out1/1
  Gain/1 -> Sum1/2
  Delay/1 -> Gain/1
  Sum1/1 -> Delay/1, GainH/1

== system Filter/HighpassH/Resonator68 ==
  In1 : Inport
  Delay : Delay  DelayLength=1
  Gain : Gain  Gain=-0.8637+0.50401i
  GainH : Gain  Gain=-0.27445-0.9616i
  Sum1 : Sum  Inputs=|++
  Out1 : Outport
  wires:
  In1/1 -> Sum1/1
  GainH/1 -> Out1/1
  Gain/1 -> Sum1/2
  Delay/1 -> Gain/1
  Sum1/1 -> Delay/1, GainH/1

== system Filter/HighpassH/Resonator69 ==
  In1 : Inport
  Delay : Delay  DelayLength=1
  Gain : Gain  Gain=-0.87738+0.4798i
  GainH : Gain  Gain=0.26106+0.96532i
  Sum1 : Sum  Inputs=|++
  Out1 : Outport
  wires:
  In1/1 -> Sum1/1
  GainH/1 -> Out1/1
  Gain/1 -> Sum1/2
  Delay/1 -> Gain/1
  Sum1/1 -> Delay/1, GainH/1

== system Filter/HighpassH/Resonator7 ==
  In1 : Inport
  Delay : Delay  DelayLength=1
  Gain : Gain  Gain=0.60784+0.79406i
  GainH : Gain  Gain=0.90269+0.4303i
  Sum1 : Sum  Inputs=|++
  Out1 : Outport
  wires:
  In1/1 -> Sum1/1
  GainH/1 -> Out1/1
  Gain/1 -> Sum1/2
  Delay/1 -> Gain/1
  Sum1/1 -> Delay/1, GainH/1

== system Filter/HighpassH/Resonator70 ==
  In1 : Inport
  Delay : Delay  DelayLength=1
  Gain : Gain  Gain=-0.89037+0.45523i
  GainH : Gain  Gain=-0.24761-0.96886i
  Sum1 : Sum  Inputs=|++
  Out1 : Outport
  wires:
  In1/1 -> Sum1/1
  GainH/1 -> Out1/1
  Gain/1 -> Sum1/2
  Delay/1 -> Gain/1
  Sum1/1 -> Delay/1, GainH/1

== system Filter/HighpassH/Resonator71 ==
  In1 : Inport
  Delay : Delay  DelayLength=1
  Gain : Gain  Gain=-0.90269+0.4303i
  GainH : Gain  Gain=0.23412+0.97221i
  Sum1 : Sum  Inputs=|++
  Out1 : Outport
  wires:
  In1/1 -> Sum1/1
  GainH/1 -> Out1/1
  Gain/1 -> Sum1/2
  Delay/1 -> Gain/1
  Sum1/1 -> Delay/1, GainH/1

== system Filter/HighpassH/Resonator72 ==
  In1 : Inport
  Delay : Delay  DelayLength=1
  Gain : Gain  Gain=-0.9143+0.40504i
  GainH : Gain  Gain=-0.22058-0.97537i
  Sum1 : Sum  Inputs=|++
  Out1 : Outport
  wires:
  In1/1 -> Sum1/1
  GainH/1 -> Out1/1
  Gain/1 -> Sum1/2
  Delay/1 -> Gain/1
  Sum1/1 -> Delay/1, GainH/1

== system Filter/HighpassH/Resonator73 ==
  In1 : Inport
  Delay : Delay  DelayLength=1
  Gain : Gain  Gain=-0.9252+0.37947i
  GainH : Gain  Gain=0.20701+0.97834i
  Sum1 : Sum  Inputs=|++
  Out1 : Outport
  wires:
  In1/1 -> Sum1/1
  GainH/1 -> Out1/1
  Gain/1 -> Sum1/2
  Delay/1 -> Gain/1
  Sum1/1 -> Delay/1, GainH/1

== system Filter/HighpassH/Resonator74 ==
  In1 : Inport
  Delay : Delay  DelayLength=1
  Gain : Gain  Gain=-0.93539+0.3536i
  GainH : Gain  Gain=-0.19339-0.98112i
  Sum1 : Sum  Inputs=|++
  Out1 : Outport
  wires:
  In1/1 -> Sum1/1
  GainH/1 -> Out1/1
  Gain/1 -> Sum1/2
  Delay/1 -> Gain/1
  Sum1/1 -> Delay/1, GainH/1

== system Filter/HighpassH/Resonator75 ==
  In1 : Inport
  Delay : Delay  DelayLength=1
  Gain : Gain  Gain=-0.94486+0.32747i
  GainH : Gain  Gain=0.17973+0.98372i
  Sum1 : Sum  Inputs=|++
  Out1 : Outport
  wires:
  In1/1 -> Sum1/1
  GainH/1 -> Out1/1
  Gain/1 -> Sum1/2
  Delay/1 -> Gain/1
  Sum1/1 -> Delay/1, GainH/1

== system Filter/HighpassH/Resonator76 ==
  In1 : Inport
  Delay : Delay  DelayLength=1
  Gain : Gain  Gain=-0.9536+0.30107i
  GainH : Gain  Gain=-0.16604-0.98612i
  Sum1 : Sum  Inputs=|++
  Out1 : Outport
  wires:
  In1/1 -> Sum1/1
  GainH/1 -> Out1/1
  Gain/1 -> Sum1/2
  Delay/1 -> Gain/1
  Sum1/1 -> Delay/1, GainH/1

== system Filter/HighpassH/Resonator77 ==
  In1 : Inport
  Delay : Delay  DelayLength=1
  Gain : Gain  Gain=-0.9616+0.27445i
  GainH : Gain  Gain=0.15231+0.98833i
  Sum1 : Sum  Inputs=|++
  Out1 : Outport
  wires:
  In1/1 -> Sum1/1
  GainH/1 -> Out1/1
  Gain/1 -> Sum1/2
  Delay/1 -> Gain/1
  Sum1/1 -> Delay/1, GainH/1

== system Filter/HighpassH/Resonator78 ==
  In1 : Inport
  Delay : Delay  DelayLength=1
  Gain : Gain  Gain=-0.96886+0.24761i
  GainH : Gain  Gain=-0.13856-0.99035i
  Sum1 : Sum  Inputs=|++
  Out1 : Outport
  wires:
  In1/1 -> Sum1/1
  GainH/1 -> Out1/1
  Gain/1 -> Sum1/2
  Delay/1 -> Gain/1
  Sum1/1 -> Delay/1, GainH/1

== system Filter/HighpassH/Resonator79 ==
  In1 : Inport
  Delay : Delay  DelayLength=1
  Gain : Gain  Gain=-0.97537+0.22058i
  GainH : Gain  Gain=0.12478+0.99218i
  Sum1 : Sum  Inputs=|++
  Out1 : Outport
  wires:
  In1/1 -> Sum1/1
  GainH/1 -> Out1/1
  Gain/1 -> Sum1/2
  Delay/1 -> Gain/1
  Sum1/1 -> Delay/1, GainH/1

== system Filter/HighpassH/Resonator8 ==
  In1 : Inport
  Delay : Delay  DelayLength=1
  Gain : Gain  Gain=0.58553+0.81065i
  GainH : Gain  Gain=-0.89662-0.44281i
  Sum1 : Sum  Inputs=|++
  Out1 : Outport
  wires:
  In1/1 -> Sum1/1
  GainH/1 -> Out1/1
  Gain/1 -> Sum1/2
  Delay/1 -> Gain/1
  Sum1/1 -> Delay/1, GainH/1

== system Filter/HighpassH/Resonator80 ==
  In1 : Inport
  Delay : Delay  DelayLength=1
  Gain : Gain  Gain=-0.98112+0.19339i
  GainH : Gain  Gain=-0.11098-0.99382i
  Sum1 : Sum  Inputs=|++
  Out1 : Outport
  wires:
  In1/1 -> Sum1/1
  GainH/1 -> Out1/1
  Gain/1 -> Sum1/2
  Delay/1 -> Gain/1
  Sum1/1 -> Delay/1, GainH/1

== system Filter/HighpassH/Resonator81 ==
  In1 : Inport
  Delay : Delay  DelayLength=1
  Gain : Gain  Gain=-0.98612+0.16604i
  GainH : Gain  Gain=0.097152+0.99527i
  Sum1 : Sum  Inputs=|++
  Out1 : Outport
  wires:
  In1/1 -> Sum1/1
  GainH/1 -> Out1/1
  Gain/1 -> Sum1/2
  Delay/1 -> Gain/1
  Sum1/1 -> Delay/1, GainH/1

== system Filter/HighpassH/Resonator82 ==
  In1 : Inport
  Delay : Delay  DelayLength=1
  Gain : Gain  Gain=-0.99035+0.13856i
  GainH : Gain  Gain=-0.083308-0.99652i
  Sum1 : Sum  Inputs=|++
  Out1 : Outport
  wires:
  In1/1 -> Sum1/1
  GainH/1 -> Out1/1
  Gain/1 -> Sum1/2
  Delay/1 -> Gain/1
  Sum1/1 -> Delay/1, GainH/1

== system Filter/HighpassH/Resonator83 ==
  In1 : Inport
  Delay : Delay  DelayLength=1
  Gain : Gain  Gain=-0.99382+0.11098i
  GainH : Gain  Gain=0.069448+0.99759i
  Sum1 : Sum  Inputs=|++
  Out1 : Outport
  wires:
  In1/1 -> Sum1/1
  GainH/1 -> Out1/1
  Gain/1 -> Sum1/2
  Delay/1 -> Gain/1
  Sum1/1 -> Delay/1, GainH/1

== system Filter/HighpassH/Resonator84 ==
  In1 : Inport
  Delay : Delay  DelayLength=1
  Gain : Gain  Gain=-0.99652+0.083308i
  GainH : Gain  Gain=-0.055575-0.99845i
  Sum1 : Sum  Inputs=|++
  Out1 : Outport
  wires:
  In1/1 -> Sum1/1
  GainH/1 -> Out1/1
  Gain/1 -> Sum1/2
  Delay/1 -> Gain/1
  Sum1/1 -> Delay/1, GainH/1

== system Filter/HighpassH/Resonator85 ==
  In1 : Inport
  Delay : Delay  DelayLength=1
  Gain : Gain  Gain=-0.99845+0.055575i
  GainH : Gain  Gain=0.04169+0.99913i
  Sum1 : Sum  Inputs=|++
  Out1 : Outport
  wires:
  In1/1 -> Sum1/1
  GainH/1 -> Out1/1
  Gain/1 -> Sum1/2
  Delay/1 -> Gain/1
  Sum1/1 -> Delay/1, GainH/1

== system Filter/HighpassH/Resonator86 ==
  In1 : Inport
  Delay : Delay  DelayLength=1
  Gain : Gain  Gain=-0.99961+0.027798i
  GainH : Gain  Gain=-0.027798-0.99961i
  Sum1 : Sum  Inputs=|++
  Out1 : Outport
  wires:
  In1/1 -> Sum1/1
  GainH/1 -> Out1/1
  Gain/1 -> Sum1/2
  Delay/1 -> Gain/1
  Sum1/1 -> Delay/1, GainH/1

== system Filter/HighpassH/Resonator87 ==
  In1 : Inport
  Delay : Delay  DelayLength=1
  Gain : Gain  Gain=-1+1.2246e-16i
  GainH : Gain  Gain=0.0139+0.9999i
  Sum1 : Sum  Inputs=|++
  Out1 : Outport
  wires:
  In1/1 -> Sum1/1
  GainH/1 -> Out1/1
  Gain/1 -> Sum1/2
  Delay/1 -> Gain/1
  Sum1/1 -> Delay/1, GainH/1

== system Filter/HighpassH/Resonator88 ==
  In1 : Inport
  Delay : Delay  DelayLength=1
  Gain : Gain  Gain=-0.99961-0.027798i
  GainH : Gain  Gain=1.9106e-14-1i
  Sum1 : Sum  Inputs=|++
  Out1 : Outport
  wires:
  In1/1 -> Sum1/1
  GainH/1 -> Out1/1
  Gain/1 -> Sum1/2
  Delay/1 -> Gain/1
  Sum1/1 -> Delay/1, GainH/1

== system Filter/HighpassH/Resonator89 ==
  In1 : Inport
  Delay : Delay  DelayLength=1
  Gain : Gain  Gain=-0.99845-0.055575i
  GainH : Gain  Gain=0.0139-0.9999i
  Sum1 : Sum  Inputs=|++
  Out1 : Outport
  wires:
  In1/1 -> Sum1/1
  GainH/1 -> Out1/1
  Gain/1 -> Sum1/2
  Delay/1 -> Gain/1
  Sum1/1 -> Delay/1, GainH/1

== system Filter/HighpassH/Resonator9 ==
  In1 : Inport
  Delay : Delay  DelayLength=1
  Gain : Gain  Gain=0.56277+0.82661i
  GainH : Gain  Gain=0.89037+0.45523i
  Sum1 : Sum  Inputs=|++
  Out1 : Outport
  wires:
  In1/1 -> Sum1/1
  GainH/1 -> Out1/1
  Gain/1 -> Sum1/2
  Delay/1 -> Gain/1
  Sum1/1 -> Delay/1, GainH/1

== system Filter/HighpassH/Resonator90 ==
  In1 : Inport
  Delay : Delay  DelayLength=1
  Gain : Gain  Gain=-0.99652-0.083308i
  GainH : Gain  Gain=-0.027798+0.99961i
  Sum1 : Sum  Inputs=|++
  Out1 : Outport
  wires:
  In1/1 -> Sum1/1
  GainH/1 -> Out1/1
  Gain/1 -> Sum1/2
  Delay/1 -> Gain/1
  Sum1/1 -> Delay/1, GainH/1

== system Filter/HighpassH/Resonator91 ==
  In1 : Inport
  Delay : Delay  DelayLength=1
  Gain : Gain  Gain=-0.99382-0.11098i
  GainH : Gain  Gain=0.04169-0.99913i
  Sum1 : Sum  Inputs=|++
  Out1 : Outport
  wires:
  In1/1 -> Sum1/1
  GainH/1 -> Out1/1
  Gain/1 -> Sum1/2
  Delay/1 -> Gain/1
  Sum1/1 -> Delay/1, GainH/1

== system Filter/HighpassH/Resonator92 ==
  In1 : Inport
  Delay : Delay  DelayLength=1
  Gain : Gain  Gain=-0.99035-0.13856i
  GainH : Gain  Gain=-0.055575+0.99845i
  Sum1 : Sum  Inputs=|++
  Out1 : Outport
  wires:
  In1/1 -> Sum1/1
  GainH/1 -> Out1/1
  Gain/1 -> Sum1/2
  Delay/1 -> Gain/1
  Sum1/1 -> Delay/1, GainH/1

== system Filter/HighpassH/Resonator93 ==
  In1 : Inport
  Delay : Delay  DelayLength=1
  Gain : Gain  Gain=-0.98612-0.16604i
  GainH : Gain  Gain=0.069448-0.99759i
  Sum1 : Sum  Inputs=|++
  Out1 : Outport
  wires:
  In1/1 -> Sum1/1
  GainH/1 -> Out1/1
  Gain/1 -> Sum1/2
  Delay/1 -> Gain/1
  Sum1/1 -> Delay/1, GainH/1

== system Filter/HighpassH/Resonator94 ==
  In1 : Inport
  Delay : Delay  DelayLength=1
  Gain : Gain  Gain=-0.98112-0.19339i
  GainH : Gain  Gain=-0.083308+0.99652i
  Sum1 : Sum  Inputs=|++
  Out1 : Outport
  wires:
  In1/1 -> Sum1/1
  GainH/1 -> Out1/1
  Gain/1 -> Sum1/2
  Delay/1 -> Gain/1
  Sum1/1 -> Delay/1, GainH/1

== system Filter/HighpassH/Resonator95 ==
  In1 : Inport
  Delay : Delay  DelayLength=1
  Gain : Gain  Gain=-0.97537-0.22058i
  GainH : Gain  Gain=0.097152-0.99527i
  Sum1 : Sum  Inputs=|++
  Out1 : Outport
  wires:
  In1/1 -> Sum1/1
  GainH/1 -> Out1/1
  Gain/1 -> Sum1/2
  Delay/1 -> Gain/1
  Sum1/1 -> Delay/1, GainH/1

== system Filter/HighpassH/Resonator96 ==
  In1 : Inport
  Delay : Delay  DelayLength=1
  Gain : Gain  Gain=-0.96886-0.24761i
  GainH : Gain  Gain=-0.11098+0.99382i
  Sum1 : Sum  Inputs=|++
  Out1 : Outport
  wires:
  In1/1 -> Sum1/1
  GainH/1 -> Out1/1
  Gain/1 -> Sum1/2
  Delay/1 -> Gain/1
  Sum1/1 -> Delay/1, GainH/1

== system Filter/HighpassH/Resonator97 ==
  In1 : Inport
  Delay : Delay  DelayLength=1
  Gain : Gain  Gain=-0.9616-0.27445i
  GainH : Gain  Gain=0.12478-0.99218i
  Sum1 : Sum  Inputs=|++
  Out1 : Outport
  wires:
  In1/1 -> Sum1/1
  GainH/1 -> Out1/1
  Gain/1 -> Sum1/2
  Delay/1 -> Gain/1
  Sum1/1 -> Delay/1, GainH/1

== system Filter/HighpassH/Resonator98 ==
  In1 : Inport
  Delay : Delay  DelayLength=1
  Gain : Gain  Gain=-0.9536-0.30107i
  GainH : Gain  Gain=-0.13856+0.99035i
  Sum1 : Sum  Inputs=|++
  Out1 : Outport
  wires:
  In1/1 -> Sum1/1
  GainH/1 -> Out1/1
  Gain/1 -> Sum1/2
  Delay/1 -> Gain/1
  Sum1/1 -> Delay/1, GainH/1

== system Filter/HighpassH/Resonator99 ==
  In1 : Inport
  Delay : Delay  DelayLength=1
  Gain : Gain  Gain=-0.94486-0.32747i
  GainH : Gain  Gain=0.15231-0.98833i
  Sum1 : Sum  Inputs=|++
  Out1 : Outport
  wires:
  In1/1 -> Sum1/1
  GainH/1 -> Out1/1
  Gain/1 -> Sum1/2
  Delay/1 -> Gain/1
  Sum1/1 -> Delay/1, GainH/1

== system Filter/HighpassH/ResonatorTemplate ==
  In1 : Inport
  Delay : Delay  DelayLength=1
  Gain : Gain
  GainH : Gain
  Sum1 : Sum  Inputs=|++
  Out1 : Outport
  wires:
  Sum1/1 -> GainH/1, Delay/1
  Delay/1 -> Gain/1
  Gain/1 -> Sum1/2
  GainH/1 -> Out1/1
  In1/1 -> Sum1/1

== system Filter/LowpassH/Resonator1 ==
  In1 : Inport
  Delay : Delay  DelayLength=1
  Gain : Gain  Gain=0.99961+0.027798i
  GainH : Gain
  Sum1 : Sum  Inputs=|++
  Out1 : Outport
  wires:
  In1/1 -> Sum1/1
  GainH/1 -> Out1/1
  Gain/1 -> Sum1/2
  Delay/1 -> Gain/1
  Sum1/1 -> Delay/1, GainH/1

== system Filter/LowpassH/Resonator10 ==
  In1 : Inport
  Delay : Delay  DelayLength=1
  Gain : Gain  Gain=0.9616+0.27445i
  GainH : Gain  Gain=0.72887-0.68465i
  Sum1 : Sum  Inputs=|++
  Out1 : Outport
  wires:
  In1/1 -> Sum1/1
  GainH/1 -> Out1/1
  Gain/1 -> Sum1/2
  Delay/1 -> Gain/1
  Sum1/1 -> Delay/1, GainH/1

== system Filter/LowpassH/Resonator11 ==
  In1 : Inport
  Delay : Delay  DelayLength=1
  Gain : Gain  Gain=0.9536+0.30107i
  GainH : Gain  Gain=0.034745-0.9994i
  Sum1 : Sum  Inputs=|++
  Out1 : Outport
  wires:
  In1/1 -> Sum1/1
  GainH/1 -> Out1/1
  Gain/1 -> Sum1/2
  Delay/1 -> Gain/1
  Sum1/1 -> Delay/1, GainH/1

== system Filter/LowpassH/Resonator12 ==
  In1 : Inport
  Delay : Delay  DelayLength=1
  Gain : Gain  Gain=0.94486+0.32747i
  GainH : Gain  Gain=-0.67957-0.73361i
  Sum1 : Sum  Inputs=|++
  Out1 : Outport
  wires:
  In1/1 -> Sum1/1
  GainH/1 -> Out1/1
  Gain/1 -> Sum1/2
  Delay/1 -> Gain/1
  Sum1/1 -> Delay/1, GainH/1

== system Filter/LowpassH/Resonator13 ==
  In1 : Inport
  Delay : Delay  DelayLength=1
  Gain : Gain  Gain=0.9616-0.27445i
  GainH : Gain  Gain=-0.67957+0.73361i
  Sum1 : Sum  Inputs=|++
  Out1 : Outport
  wires:
  In1/1 -> Sum1/1
  GainH/1 -> Out1/1
  Gain/1 -> Sum1/2
  Delay/1 -> Gain/1
  Sum1/1 -> Delay/1, GainH/1

== system Filter/LowpassH/Resonator14 ==
  In1 : Inport
  Delay : Delay  DelayLength=1
  Gain : Gain  Gain=0.96886-0.24761i
  GainH : Gain  Gain=0.034745+0.9994i
  Sum1 : Sum  Inputs=|++
  Out1 : Outport
  wires:
  In1/1 -> Sum1/1
  GainH/1 -> Out1/1
  Gain/1 -> Sum1/2
  Delay/1 -> Gain/1
  Sum1/1 -> Delay/1, GainH/1

== system Filter/LowpassH/Resonator15 ==
  In1 : Inport
  Delay : Delay  DelayLength=1
  Gain : Gain  Gain=0.97537-0.22058i
  GainH : Gain  Gain=0.72887+0.68465i
  Sum1 : Sum  Inputs=|++
  Out1 : Outport
  wires:
  In1/1 -> Sum1/1
  GainH/1 -> Out1/1
  Gain/1 -> Sum1/2
  Delay/1 -> Gain/1
  Sum1/1 -> Delay/1, GainH/1

== system Filter/LowpassH/Resonator16 ==
  In1 : Inport
  Delay : Delay  DelayLength=1
  Gain : Gain  Gain=0.98112-0.19339i
  GainH : Gain  Gain=0.99961-0.027798i
  Sum1 : Sum  Inputs=|++
  Out1 : Outport
  wires:
  In1/1 -> Sum1/1
  GainH/1 -> Out1/1
  Gain/1 -> Sum1/2
  Delay/1 -> Gain/1
  Sum1/1 -> Delay/1, GainH/1

== system Filter/LowpassH/Resonator17 ==
  In1 : Inport
  Delay : Delay  DelayLength=1
  Gain : Gain  Gain=0.98612-0.16604i
  GainH : Gain  Gain=0.6897-0.7241i
  Sum1 : Sum  Inputs=|++
  Out1 : Outport
  wires:
  In1/1 -> Sum1/1
  GainH/1 -> Out1/1
  Gain/1 -> Sum1/2
  Delay/1 -> Gain/1
  Sum1/1 -> Delay/1, GainH/1

== system Filter/LowpassH/Resonator18 ==
  In1 : Inport
  Delay : Delay  DelayLength=1
  Gain : Gain  Gain=0.99035-0.13856i
  GainH : Gain  Gain=-0.02085-0.99978i
  Sum1 : Sum  Inputs=|++
  Out1 : Outport
  wires:
  In1/1 -> Sum1/1
  GainH/1 -> Out1/1
  Gain/1 -> Sum1/2
  Delay/1 -> Gain/1
  Sum1/1 -> Delay/1, GainH/1

== system Filter/LowpassH/Resonator19 ==
  In1 : Inport
  Delay : Delay  DelayLength=1
  Gain : Gain  Gain=0.99382-0.11098i
  GainH : Gain  Gain=-0.71929-0.69471i
  Sum1 : Sum  Inputs=|++
  Out1 : Outport
  wires:
  In1/1 -> Sum1/1
  GainH/1 -> Out1/1
  Gain/1 -> Sum1/2
  Delay/1 -> Gain/1
  Sum1/1 -> Delay/1, GainH/1

== system Filter/LowpassH/Resonator2 ==
  In1 : Inport
  Delay : Delay  DelayLength=1
  Gain : Gain  Gain=0.99845+0.055575i
  GainH : Gain  Gain=0.70956-0.70465i
  Sum1 : Sum  Inputs=|++
  Out1 : Outport
  wires:
  In1/1 -> Sum1/1
  GainH/1 -> Out1/1
  Gain/1 -> Sum1/2
  Delay/1 -> Gain/1
  Sum1/1 -> Delay/1, GainH/1

== system Filter/LowpassH/Resonator20 ==
  In1 : Inport
  Delay : Delay  DelayLength=1
  Gain : Gain  Gain=0.99652-0.083308i
  GainH : Gain  Gain=-0.9999+0.0139i
  Sum1 : Sum  Inputs=|++
  Out1 : Outport
  wires:
  In1/1 -> Sum1/1
  GainH/1 -> Out1/1
  Gain/1 -> Sum1/2
  Delay/1 -> Gain/1
  Sum1/1 -> Delay/1, GainH/1

== system Filter/LowpassH/Resonator21 ==
  In1 : Inport
  Delay : Delay  DelayLength=1
  Gain : Gain  Gain=0.99845-0.055575i
  GainH : Gain  Gain=-0.6997+0.71444i
  Sum1 : Sum  Inputs=|++
  Out1 : Outport
  wires:
  In1/1 -> Sum1/1
  GainH/1 -> Out1/1
  Gain/1 -> Sum1/2
  Delay/1 -> Gain/1
  Sum1/1 -> Delay/1, GainH/1

== system Filter/LowpassH/Resonator22 ==
  In1 : Inport
  Delay : Delay  DelayLength=1
  Gain : Gain  Gain=0.99961-0.027798i
  GainH : Gain  Gain=0.0069504+0.99998i
  Sum1 : Sum  Inputs=|++
  Out1 : Outport
  wires:
  In1/1 -> Sum1/1
  GainH/1 -> Out1/1
  Gain/1 -> Sum1/2
  Delay/1 -> Gain/1
  Sum1/1 -> Delay/1, GainH/1
